simulink model "Sim_NLBM_Train_2016"  (Simulink 8.7)
settings: Solver=ode5  SolverMode=SingleTasking  StartTime=T_str  StopTime=T_end  FixedStep=dt_cal  RelTol=1e-3  AbsTol=1e-6
values from neighbouring files (symbols this model uses):
  Bcd = Bcd/gain_snr    [ctrlr_20.m]
  CC = zeros(Num_DOF)    [Bld_NLBM.m]
  Ccd = Ccd/gain_ctr    [ctrlr_20.m]
  Dcd = Dcd/gain_snr/gain_ctr    [ctrlr_20.m]
  gain_ctr = Max_frc/Max_voltd    (= 100000)    [ctrlr_20.m]
  intensity = 1.5    [TrainFuzzy_2016.m]
  Kf = K_load*K_mult*gain_ctr    [ctrlr_20.m]
  KK = zeros(Num_DOF)    [Bld_NLBM.m]
  MM = zeros(Num_DOF)    [Bld_NLBM.m]
  SL_ctr = Max_voltd    (= 10)    [ctrlr_20.m]
  SL_snr = Max_volts    (= 10)    [ctrlr_20.m]
  ST_snr = 0.01    [ctrlr_20.m]
  Tcd = 0.01    [ctrlr_20.m]
undefined symbols (not defined in the file or in its folder): Acd
undefined symbols (not defined in the file): Ds
libraries: simulink x1
settings Model: Creator=nec1  LastModifiedBy=User
settings DataIOCC: Decimation=Num_decimate  LimitDataPoints=off  SignalLoggingSaveFormat=ModelDataLogs
settings OptimizationCC: BlockReduction=off  BooleanDataType=off  ExpressionDepthLimit=2147483647  InitFltsAndDblsToZero=on
settings DebuggingCC: SaveWithParameterizedLinksMsg=none  SignalResolutionControl=TryResolveAllWithWarning  MultiTaskDSMMsg=warning  MultiTaskCondExecSysMsg=none  FcnCallInpInsideContextMsg=EnableAllAsWarning  UnconnectedInputMsg=none  UnconnectedOutputMsg=none  UnconnectedLineMsg=none  StateNameClashWarn=warning
settings HardwareCC: TargetUnknown=on
settings RTWCC: TemplateMakefile=grt_vc.tmf
settings GRTTargetCC: TargetFcnLib=ansi_tfl_tmw.mat  GeneratePreprocessorConditionals=Use local settings  CombineOutputUpdateFcns=off  GRTInterface=on
settings ConfigComp: CovModelRefEnable=off

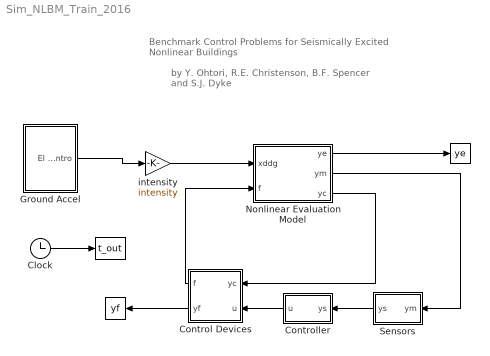
== system Sim_NLBM_Train_2016 ==
  note: by
      | Y. Ohtori, R.E. Christenson, B.F. Spencer
      | and S.J. Dyke
  note: Benchmark Control Problems
      | for Seismically Excited Nonlinear Buildings
  "  " : ToWorkspace  VariableName=ye  SampleTime=-1
      settings: Decimation=Num_decimate
  "   " : ToWorkspace  VariableName=yf  SampleTime=-1
      settings: Decimation=Num_decimate
  "    " : ToWorkspace  VariableName=t_out  SampleTime=-1
      settings: Decimation=Num_decimate
  Clock : Clock
  Control Devices : Subsystem
  Controller : Subsystem
  Ground Accel : Subsystem
  Nonlinear Evaluation Model : Subsystem
  "Sensors " : Subsystem
  intensity : Gain  Gain=intensity  SaturateOnIntegerOverflow=on  OutDataTypeStr=Inherit: Same as input  ParamDataTypeStr=Inherit: Same as input
  wires:
  intensity/1 -> Nonlinear Evaluation Model/1(xddg)
  Nonlinear Evaluation Model/1(ye) -> "  "/1
  Nonlinear Evaluation Model/2(ym) -> "Sensors "/1(ym)
  Controller/1(u) -> Control Devices/2(u)
  "Sensors "/1(ys) -> Controller/1(ys)
  Nonlinear Evaluation Model/3(yc) -> Control Devices/1(yc)
  Control Devices/2(yf) -> "   "/1
  Control Devices/1(f) -> Nonlinear Evaluation Model/2(f)
  Clock/1 -> "    "/1
  Ground Accel/1(El Centro) -> intensity/1

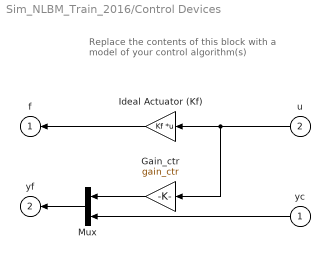
== system Sim_NLBM_Train_2016/Control Devices ==
  note: Replace the contents of this block
      | with a model of your control algorithm(s)
  yc : Inport
  u : Inport  Port=2
  Gain_ctr : Gain  Gain=gain_ctr  SaturateOnIntegerOverflow=on  OutDataTypeStr=Inherit: Same as input  ParamDataTypeStr=Inherit: Same as input
  Ideal Actuator (Kf) : Gain  Gain=Kf  Multiplication=Matrix(K*u)  SaturateOnIntegerOverflow=on  OutDataTypeStr=Inherit: Same as input  ParamDataTypeStr=Inherit: Same as input
  Mux : Mux  Inputs=2
  f : Outport  InitialOutput=0
  yf : Outport  Port=2  InitialOutput=0
  wires:
  Ideal Actuator (Kf)/1 -> f/1
  Mux/1 -> yf/1
  yc/1 -> Mux/2
  u/1 -> Ideal Actuator (Kf)/1, Gain_ctr/1
  Gain_ctr/1 -> Mux/1

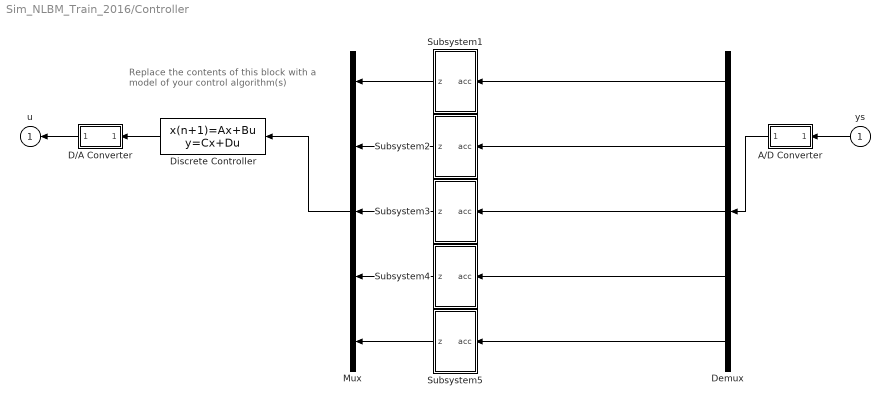
== system Sim_NLBM_Train_2016/Controller ==
  note: Replace the contents of this block
      | with a model of your control algorithm(s)
  ys : Inport
  A/D Converter : Subsystem
  D/A Converter : Subsystem
  Demux : Demux  Outputs=5
  Discrete Controller : DiscreteStateSpace  A=Acd  B=Bcd  C=Ccd  D=Dcd  SampleTime=Tcd
  Mux : Mux  Inputs=5
  Subsystem1 : Subsystem
  Subsystem2 : Subsystem
  Subsystem3 : Subsystem
  Subsystem4 : Subsystem
  Subsystem5 : Subsystem
  u : Outport  InitialOutput=0
  wires:
  ys/1 -> A/D Converter/1(y(t))
  Discrete Controller/1 -> D/A Converter/1(u(k))
  D/A Converter/1(u(t)) -> u/1
  A/D Converter/1(y(k)) -> Demux/1
  Demux/1 -> Subsystem1/1(acc)
  Mux/1 -> Discrete Controller/1
  Subsystem1/1(z) -> Mux/1
  Demux/2 -> Subsystem2/1(acc)
  Demux/3 -> Subsystem3/1(acc)
  Demux/5 -> Subsystem5/1(acc)
  Demux/4 -> Subsystem4/1(acc)
  Subsystem2/1(z) -> Mux/2
  Subsystem3/1(z) -> Mux/3
  Subsystem4/1(z) -> Mux/4
  Subsystem5/1(z) -> Mux/5

== system Sim_NLBM_Train_2016/Ground Accel ==
  El Centro_data : FromFile  FileName=elcentro.mat
  El Centro : Outport
  wires:
  El Centro_data/1 -> El Centro/1

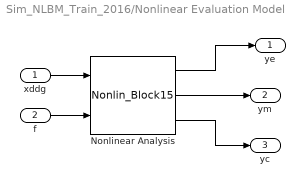
== system Sim_NLBM_Train_2016/Nonlinear Evaluation Model ==
  xddg : Inport
  f : Inport  Port=2
  Nonlinear Analysis : S-Function  FunctionName=Nonlin_Block15  Parameters=MM,CC,KK  SFunctionDeploymentMode=off  EnableBusSupport=off
  ye : Outport
  ym : Outport  Port=2
  yc : Outport  Port=3
  wires:
  xddg/1 -> Nonlinear Analysis/1
  f/1 -> Nonlinear Analysis/2
  Nonlinear Analysis/1 -> ye/1
  Nonlinear Analysis/2 -> ym/1
  Nonlinear Analysis/3 -> yc/1

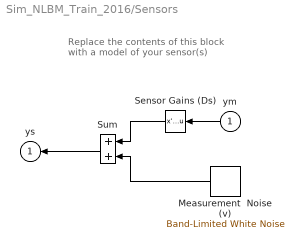
== system Sim_NLBM_Train_2016/Sensors  ==
  note: Replace the contents of this block
      | with a model of your sensor(s)
  ym : Inport
  Measurement  Noise (v) : simulink/Sources/Band-Limited White Noise  Cov=NP_snr  Ts=ST_snr  seed=Seed_snr
  Sensor Gains (Ds) : StateSpace  A=[]  B=[]  C=[]  D=K  X0=0  mask(Matrix Gain){K=Ds}
      mask prompts: K "Gain matrix:"
      mask help: Matrix Gain.
      mask Help: Multiplies input vector by entered matrix to produce output vector (y=Au).
      mask Display: disp('K')
  Sum : Sum  SaturateOnIntegerOverflow=on  InputSameDT=on  OutDataTypeStr=Inherit: Same as first input
  ys : Outport  InitialOutput=0
  wires:
  Measurement  Noise (v)/1 -> Sum/2
  Sensor Gains (Ds)/1 -> Sum/1
  ym/1 -> Sensor Gains (Ds)/1
  Sum/1 -> ys/1

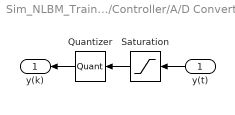
== system Sim_NLBM_Train_2016/Controller/A/D Converter ==
  y(t) : Inport
  Quantizer : Quantizer  QuantizationInterval=QI_snr
  Saturation : Saturate  UpperLimit=SL_snr  LowerLimit=-SL_snr
  y(k) : Outport
  wires:
  y(t)/1 -> Saturation/1
  Quantizer/1 -> y(k)/1
  Saturation/1 -> Quantizer/1

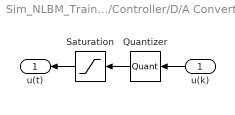
== system Sim_NLBM_Train_2016/Controller/D/A Converter ==
  u(k) : Inport
  Quantizer : Quantizer  QuantizationInterval=QI_ctr
  Saturation : Saturate  UpperLimit=SL_ctr  LowerLimit=-SL_ctr
  u(t) : Outport
  wires:
  u(k)/1 -> Quantizer/1
  Quantizer/1 -> Saturation/1
  Saturation/1 -> u(t)/1

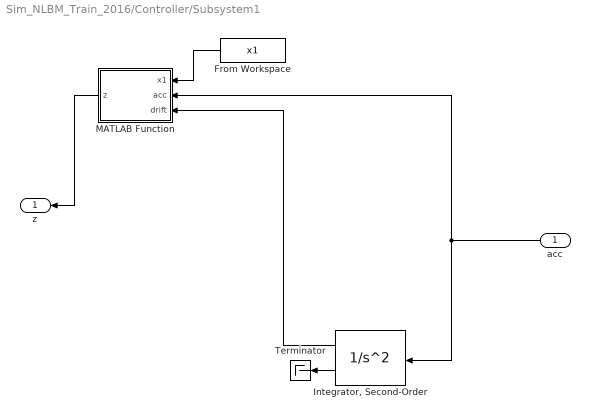
== system Sim_NLBM_Train_2016/Controller/Subsystem1 ==
  acc : Inport
  From Workspace : FromWorkspace  VariableName=x1  SampleTime=0
  "Integrator, Second-Order" : SecondOrderIntegrator
  MATLAB Function : MATLAB Function  TreatAsAtomicUnit=on
  Terminator : Terminator
  z : Outport
  wires:
  "Integrator, Second-Order"/1 -> MATLAB Function/3(drift)
  acc/1 -> MATLAB Function/2(acc), "Integrator, Second-Order"/1
  "Integrator, Second-Order"/2 -> Terminator/1
  MATLAB Function/1(z) -> z/1
  From Workspace/1 -> MATLAB Function/1(x1)

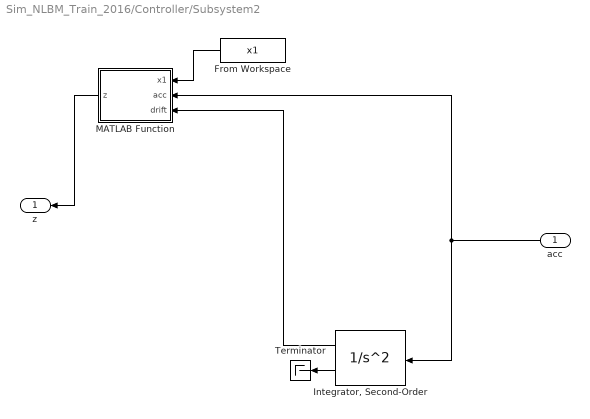
== system Sim_NLBM_Train_2016/Controller/Subsystem2 ==
  acc : Inport
  From Workspace : FromWorkspace  VariableName=x1  SampleTime=0
  "Integrator, Second-Order" : SecondOrderIntegrator
  MATLAB Function : MATLAB Function  TreatAsAtomicUnit=on
  Terminator : Terminator
  z : Outport
  wires:
  "Integrator, Second-Order"/1 -> MATLAB Function/3(drift)
  acc/1 -> MATLAB Function/2(acc), "Integrator, Second-Order"/1
  "Integrator, Second-Order"/2 -> Terminator/1
  MATLAB Function/1(z) -> z/1
  From Workspace/1 -> MATLAB Function/1(x1)

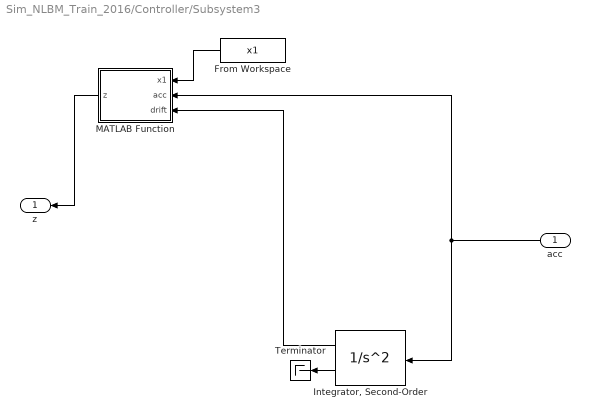
== system Sim_NLBM_Train_2016/Controller/Subsystem3 ==
  acc : Inport
  From Workspace : FromWorkspace  VariableName=x1  SampleTime=0
  "Integrator, Second-Order" : SecondOrderIntegrator
  MATLAB Function : MATLAB Function  TreatAsAtomicUnit=on
  Terminator : Terminator
  z : Outport
  wires:
  "Integrator, Second-Order"/1 -> MATLAB Function/3(drift)
  acc/1 -> MATLAB Function/2(acc), "Integrator, Second-Order"/1
  "Integrator, Second-Order"/2 -> Terminator/1
  MATLAB Function/1(z) -> z/1
  From Workspace/1 -> MATLAB Function/1(x1)

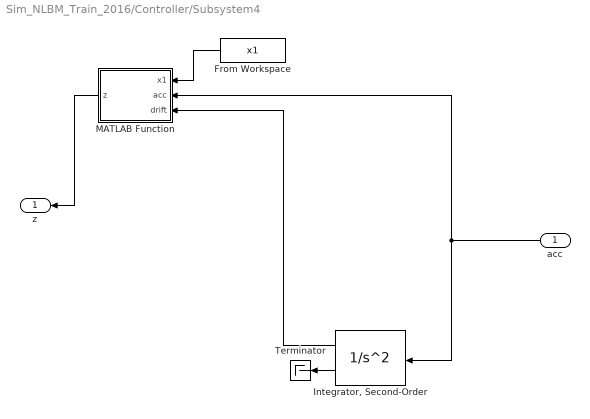
== system Sim_NLBM_Train_2016/Controller/Subsystem4 ==
  acc : Inport
  From Workspace : FromWorkspace  VariableName=x1  SampleTime=0
  "Integrator, Second-Order" : SecondOrderIntegrator
  MATLAB Function : MATLAB Function  TreatAsAtomicUnit=on
  Terminator : Terminator
  z : Outport
  wires:
  "Integrator, Second-Order"/1 -> MATLAB Function/3(drift)
  acc/1 -> MATLAB Function/2(acc), "Integrator, Second-Order"/1
  "Integrator, Second-Order"/2 -> Terminator/1
  MATLAB Function/1(z) -> z/1
  From Workspace/1 -> MATLAB Function/1(x1)

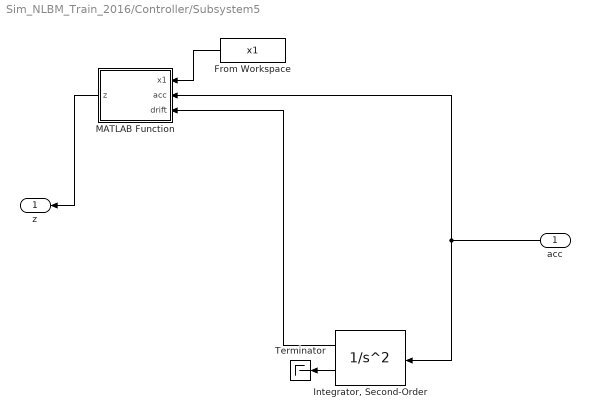
== system Sim_NLBM_Train_2016/Controller/Subsystem5 ==
  acc : Inport
  From Workspace : FromWorkspace  VariableName=x1  SampleTime=0
  "Integrator, Second-Order" : SecondOrderIntegrator
  MATLAB Function : MATLAB Function  TreatAsAtomicUnit=on
  Terminator : Terminator
  z : Outport
  wires:
  "Integrator, Second-Order"/1 -> MATLAB Function/3(drift)
  acc/1 -> MATLAB Function/2(acc), "Integrator, Second-Order"/1
  "Integrator, Second-Order"/2 -> Terminator/1
  MATLAB Function/1(z) -> z/1
  From Workspace/1 -> MATLAB Function/1(x1)

== matlab function Controller/Subsystem2/MATLAB Function ==
  data: x1 input double; acc input double; z output double; drift input double
function z = fcn(x1,acc, drift)
wA = zeros(1,5);
wB = zeros(1,5);
w = zeros(5);
zij = zeros(5);


for i = 1:5
    sigmaA = x1(2*i-1);
    cA = x1(2*i);
    if sigmaA == 0
        sigmaA = 0.5;
    end
    wA(i) = exp(-(acc-cA)^2/(2*(sigmaA)^2));
end

for j = 1:5
    sigmaB = x1(2*j+9);
    cB = x1(2*j+10);
    wB(j) = exp(-(drift-cB)^2/(2*(sigmaB)^2));
end

index = 1;
for i = 1:5
    for j = 1:5
        p = x1(20+index);
        q = x1(21+index);
        r = x1(22+index);
        index = index + 3;
        w(i,j) = wA(i)*wB(j);
        zij(i,j) = p*wA(i) + q*wB(j) + r;
    end
end

z = sum(sum(w.*zij))/sum(sum(w));
if z < 0
    z = 0;
elseif z > 10
    z = 10;
end
end

== matlab function Controller/Subsystem1/MATLAB Function ==
  data: x1 input double; acc input double; z output double; drift input double
function z = fcn(x1,acc, drift)
wA = zeros(1,5);
wB = zeros(1,5);
w = zeros(5);
zij = zeros(5);


for i = 1:5
    sigmaA = x1(2*i-1);
    cA = x1(2*i);
    if sigmaA == 0
        sigmaA = 0.5;
    end
    wA(i) = exp(-(acc-cA)^2/(2*(sigmaA)^2));
end

for j = 1:5
    sigmaB = x1(2*j+9);
    cB = x1(2*j+10);
    wB(j) = exp(-(drift-cB)^2/(2*(sigmaB)^2));
end

index = 1;
for i = 1:5
    for j = 1:5
        p = x1(20+index);
        q = x1(21+index);
        r = x1(22+index);
        index = index + 3;
        w(i,j) = wA(i)*wB(j);
        zij(i,j) = p*wA(i) + q*wB(j) + r;
    end
end

z = sum(sum(w.*zij))/sum(sum(w));
if z < 0
    z = 0;
elseif z > 10
    z = 10;
end
end

== matlab function Controller/Subsystem3/MATLAB Function ==
  data: x1 input double; acc input double; z output double; drift input double
function z = fcn(x1,acc, drift)
wA = zeros(1,5);
wB = zeros(1,5);
w = zeros(5);
zij = zeros(5);


for i = 1:5
    sigmaA = x1(2*i-1);
    cA = x1(2*i);
    if sigmaA == 0
        sigmaA = 0.5;
    end
    wA(i) = exp(-(acc-cA)^2/(2*(sigmaA)^2));
end

for j = 1:5
    sigmaB = x1(2*j+9);
    cB = x1(2*j+10);
    wB(j) = exp(-(drift-cB)^2/(2*(sigmaB)^2));
end

index = 1;
for i = 1:5
    for j = 1:5
        p = x1(20+index);
        q = x1(21+index);
        r = x1(22+index);
        index = index + 3;
        w(i,j) = wA(i)*wB(j);
        zij(i,j) = p*wA(i) + q*wB(j) + r;
    end
end

z = sum(sum(w.*zij))/sum(sum(w));
if z < 0
    z = 0;
elseif z > 10
    z = 10;
end
end

== matlab function Controller/Subsystem4/MATLAB Function ==
  data: x1 input double; acc input double; z output double; drift input double
function z = fcn(x1,acc, drift)
wA = zeros(1,5);
wB = zeros(1,5);
w = zeros(5);
zij = zeros(5);


for i = 1:5
    sigmaA = x1(2*i-1);
    cA = x1(2*i);
    if sigmaA == 0
        sigmaA = 0.5;
    end
    wA(i) = exp(-(acc-cA)^2/(2*(sigmaA)^2));
end

for j = 1:5
    sigmaB = x1(2*j+9);
    cB = x1(2*j+10);
    wB(j) = exp(-(drift-cB)^2/(2*(sigmaB)^2));
end

index = 1;
for i = 1:5
    for j = 1:5
        p = x1(20+index);
        q = x1(21+index);
        r = x1(22+index);
        index = index + 3;
        w(i,j) = wA(i)*wB(j);
        zij(i,j) = p*wA(i) + q*wB(j) + r;
    end
end

z = sum(sum(w.*zij))/sum(sum(w));
if z < 0
    z = 0;
elseif z > 10
    z = 10;
end
end

== matlab function Controller/Subsystem5/MATLAB Function ==
  data: x1 input double; acc input double; z output double; drift input double
function z = fcn(x1,acc, drift)
wA = zeros(1,5);
wB = zeros(1,5);
w = zeros(5);
zij = zeros(5);


for i = 1:5
    sigmaA = x1(2*i-1);
    cA = x1(2*i);
    if sigmaA == 0
        sigmaA = 0.5;
    end
    wA(i) = exp(-(acc-cA)^2/(2*(sigmaA)^2));
end

for j = 1:5
    sigmaB = x1(2*j+9);
    cB = x1(2*j+10);
    wB(j) = exp(-(drift-cB)^2/(2*(sigmaB)^2));
end

index = 1;
for i = 1:5
    for j = 1:5
        p = x1(20+index);
        q = x1(21+index);
        r = x1(22+index);
        index = index + 3;
        w(i,j) = wA(i)*wB(j);
        zij(i,j) = p*wA(i) + q*wB(j) + r;
    end
end

z = sum(sum(w.*zij))/sum(sum(w));
if z < 0
    z = 0;
elseif z > 10
    z = 10;
end
end
